simulink model "nmpc_traction_control_dspace"  (R2020b)
settings: Solver=ode1  StartTime=0.0  StopTime=Inf  FixedStep=0.001  RelTol=1e-3  EnableMultiTasking=on
PostLoadFcn:
  | , if any(exist('dsrtsu_mdlpostloadfcn', 'file') ~= 0), dsrtsu_mdlpostloadfcn('Execute', bdroot); end,
InitFcn:
  | , if any(exist('rtifpga_mdlclblib', 'file') ~= 0), rtifpga_mdlclblib('Init', bdroot); end,
values from neighbouring files (symbols this model uses):
  N = 4    [build_dspace.m]
  Ts = 2e-3    (= 0.002)    [build_dspace.m]
  w0 = 4.5    [build_dspace.m]
Description:
  | Standard RTI1202 template.
  | Supported MATLAB version:  R2020b.
settings Model: Tag=RTI1202  DSRTSU_INTERNAL_RTI_VER=570  DSRTSU_INTERNAL_RTI_TYPE=rti1202  RTICANMMDATA=struct('GeneralSetupData',struct('modelroot',['C:\Users\PVDC Workstation\Documents\PVDC_Project\nmpc-traction-control-forces\dspace'],'generalsettings',struct('filesettings',struct('destfolder',struct('Name','RTICANMM_FILES','Check',1),'buildfolder',struct('Name','.','Check',1),'AbsDestfolder',struct('Name',['C:\Users\PVDC Workstation\Documents\PVDC_Project\nmpc-traction-control-forces\dspace\RTICANMM_FILES']),'AbsBuildfolder',struct('Name',['C:\Users\PVDC Workstation\Documents\PVDC_Project\nmpc-traction-control-forces\dspace']))),'options',struct('addpaths',1,'rmpaths',1,'addtrcexclusion',true,'cannavigator',struct('checkmonitoring',0),'show_usrtrc',0,'use_usrtrc',0),'advanced',struct('options',ones(1,100)),'MPSetup',{{}},'RTI',struct('Type','RTI1202','Ver','7.15','Date','02-Nov-2020'),'modelname','nmpc_traction_control_dspace','block','nmpc_traction_control_dspace'))  DSRTSU_INTERNAL_RTIFPGA=170  OrderedModelArguments=off  Creator=PVDC Workstation  LastModifiedBy=PVDC Workstation
settings SolverCC: AutoInsertRateTranBlk=on  InsertRTBMode=Never (minimum delay)
settings DataIOCC: ReturnWorkspaceOutputs=off
settings OptimizationCC: BlockReduction=off  OptimizeBlockIOStorage=off  BufferReuse=off  GlobalBufferReuse=off  ExpressionFolding=off  LocalBlockOutputs=off  OptimizeDataStoreBuffers=off  BusAssignmentInplaceUpdate=off
settings DebuggingCC: PregeneratedLibrarySubsystemCodeDiagnostic=none  ArithmeticOperatorsInVariantConditions=warning
settings HardwareCC: ProdBitPerPointer=32  ProdBitPerSizeT=32  ProdBitPerPtrDiffT=32  ProdLargestAtomicInteger=Integer  ProdEndianess=BigEndian  ProdWordSize=32  ProdLongLongMode=on  ProdHWDeviceType=Custom Processor->Custom  TargetIntDivRoundTo=Zero  TargetEndianess=BigEndian  TargetHWDeviceType=Custom Processor->Custom
settings ModelReferenceCC: EnableParallelModelReferenceBuilds=on  ParallelModelReferenceMATLABWorkerInit=Load Top Model
settings SFSimCC: SimUseLocalCustomCode=off  MATLABDynamicMemAlloc=off  CustomCodeUndefinedFunction=UseInterfaceOnly
settings RTWCC: Description=dSPACE DS1202 Hardware Platform  SystemTargetFile=rti1202.tlc  MakeCommand=make_rti SKIP_TASK_CONFIGURATION=on SKIP_TASK_CONFIGURATION=on SKIP_TASK_CONFIGURATION=on SKIP_TASK_CONFIGURATION=on  TemplateMakefile=rti1202.tmf  RTWUseLocalCustomCode=off  CustomLibrary=codegen/nmpc/lib_target/libnmpc.a
settings RTWCC: CustomInclude=|
  | "./codegen"
  | "./codegen/nmpc/interface"
  | "./codegen/nmpc/lib_target"
settings RTWCC: CustomSource=|
  | codegen/nmpc/interface/nmpc_simulinkBlock.c
  | codegen/nmpc_adtool2forces.c
  | codegen/nmpc_casadi.c
settings CodeAppCC: StateflowObjectComments=on
settings STFCustomTargetCC: ParMdlRefBuildCompliant=on  ConcurrentExecutionCompliant=off  CPPClassGenCompliant=off  GRTInterface=off  SystemTargetFile=rti1202.tlc
settings GRTTargetCC: TargetLangStandard=C89/C90 (ANSI)  CompOptLevelCompliant=off  ConcurrentExecutionCompliant=off  CombineOutputUpdateFcns=off  MatFileLogging=off  CPPClassGenCompliant=off  UseToolchainInfoCompliant=off
settings ConfigComp: CovMetricSettings=dswe

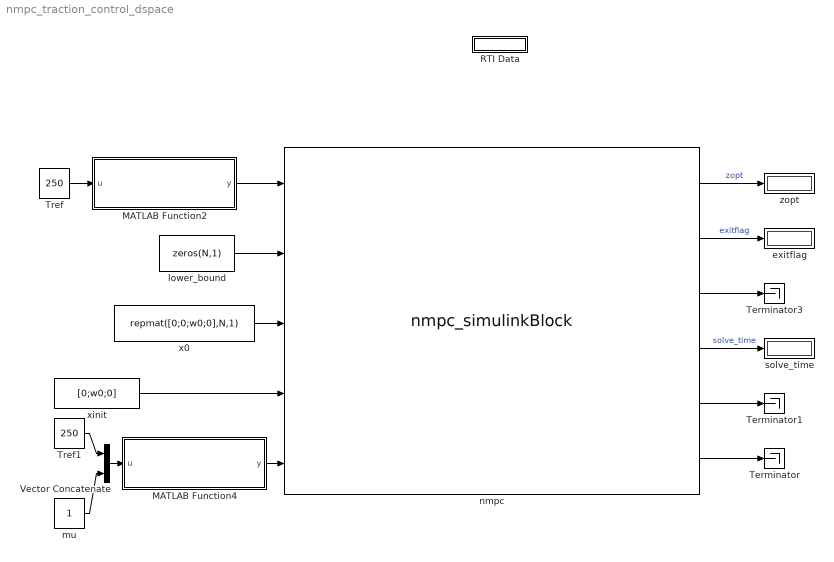
== system nmpc_traction_control_dspace ==
  MATLAB Function2 : MATLAB Function  TreatAsAtomicUnit=on
  MATLAB Function4 : MATLAB Function  TreatAsAtomicUnit=on
  RTI Data : Subsystem  Tag=struct('RTIDataServer',struct('RTIDataServerVs','2','RTIModelDescription','struct(''main'',''nmpc_traction_control_dspace'',''sub'','''',''isMp'',0)'))  LoadFcn="if exist('rtidc'), try,  rtidc('DataHostBlockClbLoad', gcbh); catch, disp(['Warning: ''LoadFcn'' for RTI Data block failed: ' lasterr]); end, end,"  mask(RTI_DATA_HOST){}
      mask help:
      | RTI Data Block.
      | This block is used by RTI to store internal model-dependent data.
      | Please keep this block on the root level of the model. Deleting this block will result in data loss.
      |
      | NEVER DELETE OR COPY THIS BLOCK!
      settings: CopyFcn="if exist('rtidc'), try,  rtidc('DataHostBlockClbCopy', gcbh); catch, disp(['Warning: ''CopyFcn'' for RTI Data block failed: ' lasterr]); end, end,"  DeleteFcn="if exist('rtidc'), try,  rtidc('DataHostBlockClbDelete', gcbh); catch, disp(['Warning: ''DeleteFcn'' for RTI Data block failed: ' lasterr]); end, end,"  ModelCloseFcn="if exist('rtidc'), try,  rtidc('DataHostBlockClbModelClose', gcbh); catch, disp(['Warning: ''ModelCloseFcn'' for RTI Data block failed: ' lasterr]); end, end,"  PreSaveFcn="if exist('rtidc'), try,  rtidc('DataHostBlockClbPreSave', gcbh); catch, disp(['Warning: ''PreSaveFcn'' for RTI Data block failed: ' lasterr]); end, end,"  PostSaveFcn="if exist('rtidc'), try,  rtidc('DataHostBlockClbPostSave', gcbh); catch, disp(['Warning: ''PostSaveFcn'' for RTI Data block failed: ' lasterr]); end, end,"  NameChangeFcn="if exist('rtidc'), try,  rtidc('DataHostBlockClbNameChange', gcbh); catch, disp(['Warning: ''NameChangeFcn'' for RTI Data block failed: ' lasterr]); end, end,"
      mask Help:
      | RTI Data Block.
      | This block is used by RTI to store internal model-dependent data.
      | Please keep this block on the root level of the model. Deleting this block will result in data loss.
      | 
      | NEVER DELETE OR COPY THIS BLOCK!
      mask Display:
      | text(0.5, 0.5, 'RTI Data', 'HorizontalAlignment', 'center');
      | plot([1 0]);
  Terminator : Terminator
  Terminator1 : Terminator
  Terminator3 : Terminator
  Tref : Constant  Value=250  SampleTime=Ts
  Tref1 : Constant  Value=250  SampleTime=Ts
  Vector Concatenate : Concatenate
  exitflag : Display
  lower_bound : Constant  Value=zeros(N,1)  SampleTime=Ts
  mu : Constant  SampleTime=Ts
  nmpc : S-Function  FunctionName=nmpc_simulinkBlock  SFunctionModules=nmpc_simulinkBlock  SFunctionDeploymentMode=off  EnableBusSupport=off  mask(nmpc_simulinkBlock){}
      mask help:
      | ---- Simulink block encapsulating your customized solver nmpc ----
      |
      | nmpc : A fast customized optimization solver.
      |
      | Copyright (C) 2013-2023 EMBOTECH AG [info@embotech.com]. All rights reserved.
      |
      |
      | This program is distributed in the hope that it will be useful.
      | EMBOTECH makes NO WARRANTIES with respect to the use of the software
      | without even the implied warranty of MERCHANTABILITY or FITNESS FOR A
      | PARTICULAR PURPOSE.
      |
      | EMBOTECH shall not have any liability for any damage arising from the use
      | of the software.
      |
      | This Agreement shall exclusively be governed by and interpreted in
      | accordance with the laws of Switzerland, excluding its principles
      | of conflict of laws. The Courts of Zurich-City shall have exclusive
      | jurisdiction in case of any dispute.
      mask Help:
      | nmpc_simulinkBlock provides an easy Simulink interface for simulating your customized solver.
      | 
      | OUTPUTS = nmpc(INPUTS) solves an optimization problem where:
      | 
      | INPUTS:
      |  - hu - matrix of size [4x1]
      |    - hl - matrix of size [4x1]
      |    - x0 - matrix of size [16x1]
      |    - xinit - matrix of size [3x1]
      |    - all_parameters - matrix of size [8x1]
      | 
      | OUTPUTS:
      |  - zopt - column vector of length 16
      |    - exitflag - scalar: (1) Optimal solution has been found (subject to desired accuracy); (0) Maximum number of interior point iterations reached; (-7) Line search could not progress
      |    - iterations - iteration number
      |    - solve_time - total solve time
      |    - primal_obj - primal objective
      |    - solver_id - solver ID of FORCESPRO solver
      | 
      |  For more information, see https://forces.embotech.com/Documentation/simulink_interface/index.html
      mask Display:
      | port_label('input', 1, 'hu')
      |   port_label('input', 2, 'hl')
      |   port_label('input', 3, 'x0')
      |   port_label('input', 4, 'xinit')
      |   port_label('input', 5, 'all_parameters')
      |   port_label('output', 1, 'zopt')
      |   port_label('output', 2, 'exitflag')
      |   port_label('output', 3, 'iterations')
      |   port_label('output', 4, 'solve_time')
      |   port_label('output', 5, 'primal_obj')
      |   port_label('output', 6, 'solver_id')
      |   if( exist('FORCES_PRO_Logo.jpg','file') ), image(imread('FORCES_PRO_Logo.jpg'),'center','on'); elseif( exist(['interface',filesep,'FORCES_PRO_Logo.jpg'],'file') ), image(imread(['interface',filesep,'FORCES_PRO_Logo.jpg']),'center','on'); elseif( exist(['nmpc',filesep,'interface',filesep,'FORCES_PRO_Logo.jpg'],'file') ), image(imread(['nmpc',filesep,'interface',filesep,'FORCES_PRO_Logo.jpg']),'center','on'); end
  solve_time : Display
  x0 : Constant  Value=repmat([0;0;w0;0],N,1)  SampleTime=Ts
  xinit : Constant  Value=[0;w0;0]  SampleTime=Ts
  zopt : Display
  wires:
  nmpc/6 -> Terminator/1
  nmpc/5 -> Terminator1/1
  nmpc/4 -> solve_time/1  "solve_time"
  nmpc/3 -> Terminator3/1
  nmpc/2 -> exitflag/1  "exitflag"
  nmpc/1 -> zopt/1  "zopt"
  MATLAB Function2/1(y) -> nmpc/1
  lower_bound/1 -> nmpc/2
  Tref1/1 -> Vector Concatenate/1
  Vector Concatenate/1 -> MATLAB Function4/1(u)
  mu/1 -> Vector Concatenate/2
  MATLAB Function4/1(y) -> nmpc/5
  Tref/1 -> MATLAB Function2/1(u)
  xinit/1 -> nmpc/4
  x0/1 -> nmpc/3

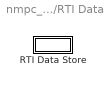
== system nmpc_traction_control_dspace/RTI Data ==
  RTI Data Store : Subsystem  Tag="struct('private',struct('version',struct('dsVer',uint32(2)),'access',struct('modified',['13-Feb-2024 15:35:04'],'type','Model','isPerm',1)),'public',struct('main',struct('data',[]),'sub',struct('name',{{'nmpc_traction_control_dspace'}},'data',{{struct('TH',struct('thTaskInfo',struct('taskType',{'TIMER','HWINT','TMRINT','SWINT','GLINT'},'tasksNumOf',{2,0,0,0,0},'srcIds',{{'TIMERA','TIMERA2'},{},{},{},{}},'taskNames',{{['Timer Task 1'],['Timer Task 2']},{},{},{},{}})),'th_tc',struct('dataType',{'TASK','TASK'},'taskGroupId',{'',''},'taskGroupList',{{},{}},'taskSchedulingPolicy',{'FCFS','FCFS'},'taskType',{'TIMER','TIMER'},'blkh',{-1,-1},'srcId',{'TIMERA','TIMERA2'},'srcSgnName',{['Timer A interrupt'],['Timer Task 1']},'srcCpuName',{'',''},'taskName',{['Timer Task 1  [0.001] s'],['Timer Task 2  [0.002] s']},'taskNameDisplayExt',{'',''},'smplTime',{0.001,0.002},'smplTimeOffs',{0,0},'hasFixedPriority',{0,0},'priority',{1,2},'hasFixedOvc',{0,0},'ovcType',{1,1},'ovcMax',{1,1}),'tc_th',struct('dataType',{'TASK','TASK'},'taskGroupId',{'',''},'taskGroupList',{{},{}},'taskSchedulingPolicy',{'FCFS','FCFS'},'taskType',{'TIMER','TIMER'},'blkh',{-1,-1},'srcId',{'TIMERA','TIMERA2'},'srcSgnName',{['Timer A interrupt'],['Timer Task 1']},'srcCpuName',{'',''},'taskName',{['Timer Task 1  [0.001] s'],['Timer Task 2  [0.002] s']},'taskNameDisplayExt',{'',''},'smplTime',{0.001,0.002},'smplTimeOffs',{0,0},'hasFixedPriority',{0,0},'priority',{1,2},'hasFixedOvc',{0,0},'ovcType',{1,1},'ovcMax',{1,1}))}})))"  mask(RTI_DATA_STORE){}
      mask help:
      | RTI Data Store Block. This block is used by RTI to store internal model dependent data. Deleting this block will result in data loss.
      |
      | NEVER DELETE, COPY, OR MODIFY THIS BLOCK!
      mask Help:
      | RTI Data Store Block. This block is used by RTI to store internal model dependent data. Deleting this block will result in data loss.
      | 
      | NEVER DELETE, COPY, OR MODIFY THIS BLOCK!
      mask Display: text(0.5, 0.5, ' ', 'HorizontalAlignment', 'center');

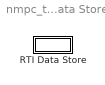
== system nmpc_traction_control_dspace/RTI Data/RTI Data Store ==
  RTI Data Store : Subsystem  mask(RTI_DATA_STORE){}
      mask help:
      | RTI Data Store Block. This block is used by RTI to store internal model dependent data. Deleting this block will result in data loss.
      |
      | NEVER DELETE, COPY, OR MODIFY THIS BLOCK!
      mask Help:
      | RTI Data Store Block. This block is used by RTI to store internal model dependent data. Deleting this block will result in data loss.
      | 
      | NEVER DELETE, COPY, OR MODIFY THIS BLOCK!
      mask Display: text(0.5, 0.5, ' ', 'HorizontalAlignment', 'center');

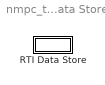
== system nmpc_traction_control_dspace/RTI Data/RTI Data Store/RTI Data Store ==
  RTI Data Store : Subsystem  mask(RTI_DATA_STORE){}
      mask help:
      | RTI Data Store Block. This block is used by RTI to store internal model dependent data. Deleting this block will result in data loss.
      |
      | NEVER DELETE, COPY, OR MODIFY THIS BLOCK!
      mask Help:
      | RTI Data Store Block. This block is used by RTI to store internal model dependent data. Deleting this block will result in data loss.
      | 
      | NEVER DELETE, COPY, OR MODIFY THIS BLOCK!
      mask Display: text(0.5, 0.5, ' ', 'HorizontalAlignment', 'center');

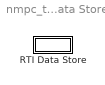
== system nmpc_traction_control_dspace/RTI Data/RTI Data Store/RTI Data Store/RTI Data Store ==
  RTI Data Store : Subsystem  mask(RTI_DATA_STORE){}
      mask help:
      | RTI Data Store Block. This block is used by RTI to store internal model dependent data. Deleting this block will result in data loss.
      |
      | NEVER DELETE, COPY, OR MODIFY THIS BLOCK!
      mask Help:
      | RTI Data Store Block. This block is used by RTI to store internal model dependent data. Deleting this block will result in data loss.
      | 
      | NEVER DELETE, COPY, OR MODIFY THIS BLOCK!
      mask Display: text(0.5, 0.5, ' ', 'HorizontalAlignment', 'center');

== system nmpc_traction_control_dspace/RTI Data/RTI Data Store/RTI Data Store/RTI Data Store/RTI Data Store ==

== matlab function nmpc_traction_control_dspace/MATLAB Function4 ==
  data: u input; y output; N parameter
function y = repeat_elements(u, N)
    y = repmat(u,N,1);
end

== matlab function nmpc_traction_control_dspace/MATLAB Function2 ==
  data: u input; y output; N parameter
function y = repeat_elements(u, N)
    y = repmat(u,N,1);
end
